simulink model "三相系统_小电流接地分析"  (R2017b)
settings: Solver=FixedStepAuto  StartTime=0.0  StopTime=1  MaxStep=1e-4  RelTol=1e-3
libraries: powerlib x17, powerlib_meascontrol x1
settings Model: Creator=wai1  LastModifiedBy=wai1
settings DebuggingCC: UnconnectedInputMsg=none  UnconnectedOutputMsg=none  UnconnectedLineMsg=none

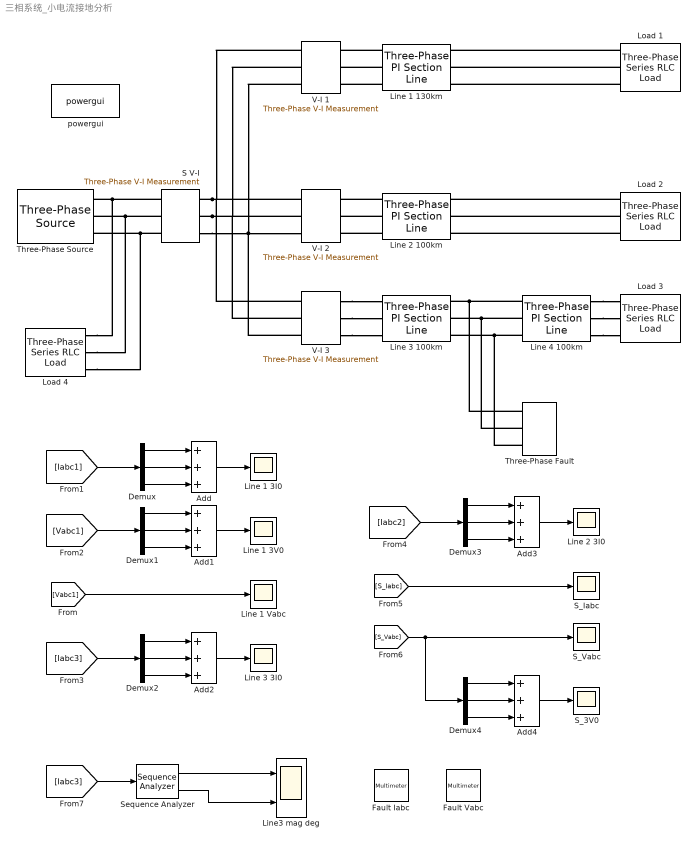
== system 三相系统_小电流接地分析 ==
  Add{,1..4} (5 alike) : Sum  Inputs=+++
  Demux{,1..4} (5 alike) : Demux  Outputs=3
  Fault Iabc : powerlib/Measurements/Multimeter  PhasorSimulation=off  OutputType=Complex  sel=[4 5 6]  L=6  Gain=[1 1 1]  yselected={'Ib: Three-Phase Fault/Fault A','Ib: Three-Phase Fault/Fault B','Ib: Three-Phase Fault/Fault C'};  PSBOutputType=1  PSBequivalent=0  AxesSetting=[0,0.1,-100,100]  Display=1  SavedBlockNames=-11
  Fault Vabc : powerlib/Measurements/Multimeter  PhasorSimulation=off  OutputType=Complex  sel=[1 2 3]  L=6  Gain=[1 1 1]  yselected={'Ub: Three-Phase Fault/Fault A','Ub: Three-Phase Fault/Fault B','Ub: Three-Phase Fault/Fault C'};  PSBOutputType=1  PSBequivalent=0  AxesSetting=[0,0.1,-100,100]  Display=1  SavedBlockNames=-11
  Line 1 130km : powerlib/Elements/Three-Phase PI Section Line  LConnTagsString=a|b|c  RConnTagsString=A|B|C  Frequency=50  Resistances=[ 0.01273 0.3864]  Inductances="[ 0.9337e-3  4.1264e-3]"  Capacitances=[12.74e-9 7.751e-9]  Length=130
      settings: SourceProductName=Simscape Power Systems
  Line 1 3I0 : Scope
  Line 1 3V0 : Scope
  Line 1 Vabc : Scope
  Line 2 100km : powerlib/Elements/Three-Phase PI Section Line  LConnTagsString=a|b|c  RConnTagsString=A|B|C  Frequency=50  Resistances=[ 0.01273 0.3864]  Inductances="[ 0.9337e-3  4.1264e-3]"  Capacitances=[12.74e-9 7.751e-9]  Length=100
      settings: SourceProductName=Simscape Power Systems
  Line 2 3I0 : Scope
  Line 3 100km : powerlib/Elements/Three-Phase PI Section Line  LConnTagsString=a|b|c  RConnTagsString=A|B|C  Frequency=50  Resistances=[ 0.01273 0.3864]  Inductances="[ 0.9337e-3  4.1264e-3]"  Capacitances=[12.74e-9 7.751e-9]  Length=100
      settings: SourceProductName=Simscape Power Systems
  Line 3 3I0 : Scope
  Line 4 100km : powerlib/Elements/Three-Phase PI Section Line  LConnTagsString=a|b|c  RConnTagsString=A|B|C  Frequency=50  Resistances=[ 0.01273 0.3864]  Inductances="[ 0.9337e-3  4.1264e-3]"  Capacitances=[12.74e-9 7.751e-9]  Length=100
      settings: SourceProductName=Simscape Power Systems
  Line3 mag deg : Scope  NumInputPorts=2
  Load 1 : powerlib/Elements/Three-Phase Series RLC Load  LConnTagsString=A|B|C  Configuration=Y (floating)  NominalVoltage=10e3  Vabc=[1e3 1e3 1e3]  Vabcp=[1e3 1e3 1e3]  NominalFrequency=50  UnbalancedPower=off  ActivePower=1.0e6  InductivePower=0.4e6  CapacitivePower=0  Pabc=[10e3 9e3 11e3]  QLabc=[100 90 110]  QCabc=[100 90 110]  Pabcp=[10e3 9e3 11e3]  QLabcp=[100 90 110]  QCabcp=[100 90 110]  Measurements=None  LoadType=constant I
  Load 2 : powerlib/Elements/Three-Phase Series RLC Load  LConnTagsString=A|B|C  Configuration=Y (grounded)  NominalVoltage=25e3  Vabc=[1e3 1e3 1e3]  Vabcp=[1e3 1e3 1e3]  NominalFrequency=50  UnbalancedPower=off  ActivePower=10e6  InductivePower=0  CapacitivePower=0  Pabc=[10e3 9e3 11e3]  QLabc=[100 90 110]  QCabc=[100 90 110]  Pabcp=[10e3 9e3 11e3]  QLabcp=[100 90 110]  QCabcp=[100 90 110]  Measurements=None  LoadType=constant I
  Load 3 : powerlib/Elements/Three-Phase Series RLC Load  LConnTagsString=A|B|C  Configuration=Y (grounded)  NominalVoltage=25e3  Vabc=[1e3 1e3 1e3]  Vabcp=[1e3 1e3 1e3]  NominalFrequency=50  UnbalancedPower=off  ActivePower=10e6  InductivePower=0  CapacitivePower=0  Pabc=[10e3 9e3 11e3]  QLabc=[100 90 110]  QCabc=[100 90 110]  Pabcp=[10e3 9e3 11e3]  QLabcp=[100 90 110]  QCabcp=[100 90 110]  Measurements=None  LoadType=constant I
  Load 4 : powerlib/Elements/Three-Phase Series RLC Load  LConnTagsString=A|B|C  Configuration=Y (floating)  NominalVoltage=10e3  Vabc=[1e3 1e3 1e3]  Vabcp=[1e3 1e3 1e3]  NominalFrequency=50  UnbalancedPower=off  ActivePower=5e6  InductivePower=0  CapacitivePower=0  Pabc=[10e3 9e3 11e3]  QLabc=[100 90 110]  QCabc=[100 90 110]  Pabcp=[10e3 9e3 11e3]  QLabcp=[100 90 110]  QCabcp=[100 90 110]  Measurements=None  LoadType=constant I
  "S V-I " : powerlib/Measurements/Three-Phase V-I Measurement  VoltageMeasurement=phase-to-ground  SetLabelV=on  LabelV=S_Vabc  Vpu=off  VpuLL=off  CurrentMeasurement=yes  SetLabelI=on  LabelI=S_Iabc  Ipu=off  Pbase=100e6  Vbase=500e3  OutputType=Complex  PhasorSimulation=off  PSBequivalent=0
  S_3V0 : Scope
  S_Iabc : Scope
  S_Vabc : Scope
  Sequence Analyzer : powerlib_meascontrol/Measurements/Sequence Analyzer  Freq=50  n=1  seq=Positive Negative Zero  InInit=[1, 0]  Ts=0
      settings: SourceProductName=Simscape Power Systems  SourceProductBaseCode=PS
  Three-Phase Fault : powerlib/Elements/Three-Phase Fault  InitialStates=0  FaultA=on  FaultB=off  FaultC=off  GroundFault=on  SwitchTimes="[0.1  0.3]"  External=off  SwitchStatus=NaN  FaultResistance=0.001  GroundResistance=0.001  SnubberResistance=1e6  SnubberCapacitance=inf  Measurements=Fault voltages and currents
  Three-Phase Source : powerlib/Electrical Sources/Three-Phase Source  InternalConnection=Y  VoltagePhases=off  Voltage=10.5e3  PhaseAngle=0  Voltage_phases=[25e3 25e3 25e3]/sqrt(3)  PhaseAngles_phases=[0 -120 +120]  Frequency=50  NonIdealSource=on  SpecifyImpedance=off  Resistance=0.009  Inductance=16.58e-5  ShortCircuitLevel=100e6  BaseVoltage=10.5e3  XRratio=7  BusType=swing  Pref=10e3  Qref=0  Prefabc=[10e3, 10e3, 10e3]  Qrefabc=[0, 0, 0]  Qmin=-inf  Qmax=inf
  V-I 1 : powerlib/Measurements/Three-Phase V-I Measurement  VoltageMeasurement=phase-to-ground  SetLabelV=on  LabelV=Vabc1  Vpu=off  VpuLL=off  CurrentMeasurement=yes  SetLabelI=on  LabelI=Iabc1  Ipu=off  Pbase=100e6  Vbase=500e3  OutputType=Complex  PhasorSimulation=off  PSBequivalent=0
  V-I 2 : powerlib/Measurements/Three-Phase V-I Measurement  VoltageMeasurement=phase-to-ground  SetLabelV=on  LabelV=Vabc2  Vpu=off  VpuLL=off  CurrentMeasurement=yes  SetLabelI=on  LabelI=Iabc2  Ipu=off  Pbase=100e6  Vbase=500e3  OutputType=Complex  PhasorSimulation=off  PSBequivalent=0
  V-I 3 : powerlib/Measurements/Three-Phase V-I Measurement  VoltageMeasurement=phase-to-ground  SetLabelV=on  LabelV=Vabc3  Vpu=off  VpuLL=off  CurrentMeasurement=yes  SetLabelI=on  LabelI=Iabc3  Ipu=off  Pbase=100e6  Vbase=500e3  OutputType=Complex  PhasorSimulation=off  PSBequivalent=0
  powergui : powerlib/powergui  Priority=1  SimulationMode=Discrete  SampleTime=50e-6  frequency=60  Iterations=50  frequencyindice=50  Pbase=100e6  ErrMax=1e-4  UnitsV=kV  UnitsW=MW  buscounter=0  FunctionMessages=off  echomessages=off  EnableUseOfTLC=off  CurrentSourceSwitches=off  DisableSnubberDevices=off  DisableRonSwitches=off  DisableVfSwitches=off  DisplayEquations=off  SolverType=Tustin/Backward Euler (TBE)  Interpol=off  ExternalGateDelay=off  methode=off  Ts=100  x0status=blocks  SPID=off  SwTol=0  HookPort=off  RestoreLinks=warning  ResistiveCurrentMeasurement=off  Frange=[0:2:500]  Ylog=off  Xlog=on  ShowGrid=off  save=off  variable=ZData  structure=0  ZoomFFT=off  StartTime=0.0  cycles=1  DisplayStyle=1  fundamental=60  FreqAxis=off  MaxFrequency=1000  frequencyindicesteady=1  RmsSteady=1  display=off
  wires:
  [Iabc1] -> Demux/1
  [Vabc1] -> Line 1 Vabc/1
  Demux/1 -> Add/1
  Demux/2 -> Add/2
  Demux/3 -> Add/3
  Add/1 -> Line 1 3I0/1
  Add1/1 -> Line 1 3V0/1
  Demux1/3 -> Add1/3
  Demux1/2 -> Add1/2
  Demux1/1 -> Add1/1
  [Vabc1] -> Demux1/1
  [Iabc3] -> Demux2/1
  Add2/1 -> Line 3 3I0/1
  Demux2/2 -> Add2/2
  Demux2/1 -> Add2/1
  Demux2/3 -> Add2/3
  Add3/1 -> Line 2 3I0/1
  Demux3/1 -> Add3/1
  [Iabc2] -> Demux3/1
  Demux3/3 -> Add3/3
  Demux3/2 -> Add3/2
  [S_Iabc] -> S_Iabc/1
  Demux4/2 -> Add4/2
  Add4/1 -> S_3V0/1
  Demux4/3 -> Add4/3
  Demux4/1 -> Add4/1
  [S_Vabc] -> Demux4/1, S_Vabc/1
  [Iabc3] -> Sequence Analyzer/1
  Sequence Analyzer/2 -> Line3 mag deg/2
  Sequence Analyzer/1 -> Line3 mag deg/1
  connections:
  "S V-I "/LConn3 -- Load 4/LConn3 -- Three-Phase Source/RConn3
  "S V-I "/LConn2 -- Load 4/LConn2 -- Three-Phase Source/RConn2
  "S V-I "/LConn1 -- Load 4/LConn1 -- Three-Phase Source/RConn1
  "S V-I "/RConn2 -- V-I 3/LConn2 -- V-I 2/LConn2 -- V-I 1/LConn2
  "S V-I "/RConn3 -- V-I 3/LConn3 -- V-I 2/LConn3 -- V-I 1/LConn3
  "S V-I "/RConn1 -- V-I 3/LConn1 -- V-I 2/LConn1 -- V-I 1/LConn1
  Line 1 130km/LConn1 -- V-I 1/RConn1
  Line 1 130km/LConn2 -- V-I 1/RConn2
  Line 1 130km/LConn3 -- V-I 1/RConn3
  Load 1/LConn1 -- Line 1 130km/RConn1
  Load 1/LConn2 -- Line 1 130km/RConn2
  Load 1/LConn3 -- Line 1 130km/RConn3
  Line 2 100km/LConn1 -- V-I 2/RConn1
  Line 2 100km/LConn2 -- V-I 2/RConn2
  Line 2 100km/LConn3 -- V-I 2/RConn3
  Load 2/LConn2 -- Line 2 100km/RConn2
  Load 2/LConn3 -- Line 2 100km/RConn3
  Load 2/LConn1 -- Line 2 100km/RConn1
  Line 4 100km/LConn2 -- Three-Phase Fault/LConn2 -- Line 3 100km/RConn2
  Line 4 100km/LConn1 -- Three-Phase Fault/LConn1 -- Line 3 100km/RConn1
  Line 4 100km/LConn3 -- Three-Phase Fault/LConn3 -- Line 3 100km/RConn3
  Line 4 100km/RConn3 -- Load 3/LConn3
  Line 4 100km/RConn2 -- Load 3/LConn2
  Line 4 100km/RConn1 -- Load 3/LConn1
  V-I 3/RConn3 -- Line 3 100km/LConn3
  V-I 3/RConn2 -- Line 3 100km/LConn2
  V-I 3/RConn1 -- Line 3 100km/LConn1
